simulink model "model1"  (R2016a)
settings: Solver=ode4  StartTime=0.0  StopTime=100  FixedStep=0.01  RelTol=1e-3
settings Model: Creator=ka28161  LastModifiedBy=ka28161

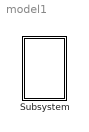
== system model1 ==
  Subsystem : Subsystem  mask{g=10, l=3, k=1, m=10, fi0=90}

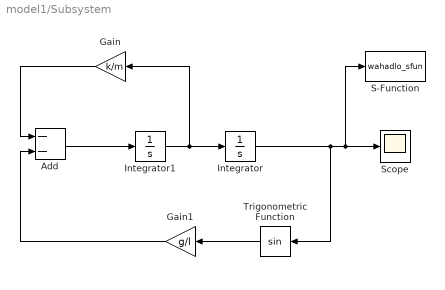
== system model1/Subsystem ==
  Add : Sum  Inputs=--
  Gain : Gain  Gain=k/m
  Gain1 : Gain  Gain=g/l
  Integrator : Integrator  InitialCondition=fi0 * pi / 180
  Integrator1 : Integrator
  S-Function : S-Function  FunctionName=wahadlo_sfun  Parameters=l, m, fi0  SFunctionDeploymentMode=off  EnableBusSupport=off
  Scope : Scope
  Trigonometric Function : Trigonometry
  wires:
  Gain/1 -> Add/1
  Integrator/1 -> S-Function/1, Scope/1, Trigonometric Function/1
  Integrator1/1 -> Gain/1, Integrator/1
  Add/1 -> Integrator1/1
  Trigonometric Function/1 -> Gain1/1
  Gain1/1 -> Add/2
